simulink model "design_observer"  (R2019a)
settings: Solver=VariableStepAuto  StartTime=0.0  StopTime=10.0  RelTol=1e-3
values from neighbouring files (symbols this model uses):
  CPrime = [CId; eye(size(AId,1))]    [regulator_2_control.m]
  DPrime = [DId; zeros(size(AId,1),1)]    [regulator_2_control.m]
  pulseAmplitude = 1    [observer_2_control.m]    (also in regulator_2_control.m)
  pulseDuration = 5    [observer_2_control.m]    (also in regulator_2_control.m)
  pulseStart = 5    [observer_2_control.m]    (also in regulator_2_control.m)
  xSelector = xSelector(2:end,:)    [regulator_2_control.m]
  ySelector = [1 zeros(1,size(AId,1))]    [regulator_2_control.m]
undefined symbols (not defined in the file or in its folder): AId, BId, TsId
settings Model: Creator=josea  LastModifiedBy=josea

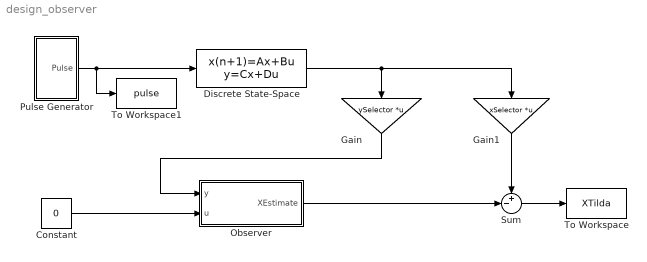
== system design_observer ==
  Constant : Constant  Value=0
  Discrete State-Space : DiscreteStateSpace  A=AId  B=BId  C=CPrime  D=DPrime  SampleTime=TsId
  Gain : Gain  Gain=ySelector  Multiplication=Matrix(K*u)
  Gain1 : Gain  Gain=xSelector  Multiplication=Matrix(K*u)
  Observer : Subsystem
  Pulse Generator : Subsystem
  Sum : Sum  Inputs=+-|
  To Workspace : ToWorkspace  VariableName=XTilda  SaveFormat=Timeseries  SampleTime=-1
  To Workspace1 : ToWorkspace  VariableName=pulse  SampleTime=-1
  wires:
  Pulse Generator/1(Pulse) -> Discrete State-Space/1, To Workspace1/1
  Discrete State-Space/1 -> Gain/1, Gain1/1
  Constant/1 -> Observer/2(u)
  Gain1/1 -> Sum/1
  Gain/1 -> Observer/1(y)
  Observer/1(XEstimate) -> Sum/2
  Sum/1 -> To Workspace/1

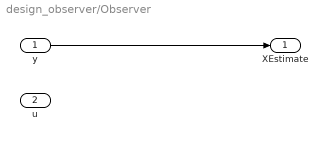
== system design_observer/Observer ==
  y : Inport
  u : Inport  Port=2
  XEstimate : Outport
  wires:
  y/1 -> XEstimate/1

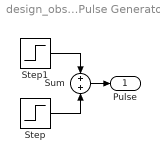
== system design_observer/Pulse Generator ==
  Step : Step  Time=pulseStart  After=pulseAmplitude  SampleTime=TsId
  Step1 : Step  Time=pulseStart+pulseDuration  After=-pulseAmplitude  SampleTime=TsId
  Sum : Sum  Inputs=+|+
  Pulse : Outport
  wires:
  Step/1 -> Sum/2
  Step1/1 -> Sum/1
  Sum/1 -> Pulse/1
